simulink model "bh_explore_1dof_Newton_vs_Simscape"  (R2026b)
settings: Solver=ode15s  StopTime=30  MaxStep=0.001  RelTol=1e-5  EnableMultiTasking=on
undefined symbols (not defined in the file or in its folder): plant_T
settings Model: Creator=smiller  LastModifiedBy=bhorton
settings SolverCC: ZeroCrossAlgorithm=Adaptive
settings DataIOCC: LimitDataPoints=on  ReturnWorkspaceOutputs=off  SaveFormat=Array
settings OptimizationCC: LifeSpan=inf
settings DebuggingCC: AllowSymbolicDim=off  ArithmeticOperatorsInVariantConditions=warning  MergeDetectMultiDrivingBlocksExec=none  SFExecutionAtInitializationDiag=none  SFNoUnconditionalDefaultTransitionDiag=warning  SFUnexpectedBacktrackingDiag=warning  SolverPrmCheckMsg=warning  StateNameClashWarn=warning  UnderspecifiedInitializationDetection=Classic
settings HardwareCC: ProdEndianess=Unspecified  ProdHWDeviceType=32-bit Generic  ProdIntDivRoundTo=Undefined  ProdLargestAtomicFloat=None
settings ModelReferenceCC: PropagateSignalLabelsOutOfModel=off
settings SFSimCC: CustomCodeUndefinedFunction=UseInterfaceOnly  SimUseLocalCustomCode=off
settings RTWCC: DLArmComputeVersion=19.05  RTWUseLocalCustomCode=off
settings CodeAppCC: StateflowObjectComments=on
settings GRTTargetCC: TargetLangStandard=C89/C90 (ANSI)
settings ConfigComp: CovExternalEMLEnable=off  CovSFcnEnable=off  CovSaveCumulativeToWorkspaceVar=on  CovSaveSingleToWorkspaceVar=on
settings SimscapeCC: SimscapeNormalizeSystem=off  SimscapeUseEnergyAccounting=off
settings ExplorerConfigSet: InternalSimMechanicsExplorerSettings=|
  | <ExplorerConfiguration>
  | 
  |   <canonicalview>planar_xy</canonicalview>
  | 
  |   <TilePanel>
  |     <TileInfo>
  |       <Tiles Columns="2" Count="2" Height="500" Rows="1" Width="911">
  |         <Row Weight="1"/>
  |         <Column Weight="0.5"/>
  |         <Column Weight="0.5"/>
  |         <Tile Height="1" Width="1" X="0" Y="0"/>
  |         <Tile Height="1" Width="1" X="1" Y="0"/>
  |       </Tiles>
  |     </TileInfo>
  |     <SceneInfo>
  |       <SceneViewer>
  |         <IsThisViewStd>
  |           <IsStandardView>off</IsStandardView>
  |           <StandardViewName>Front</StandardViewName>
  |         </IsThisViewStd>
  |         <BGColor>
  |           <R>0.60000002384185791</R>
  |           <G>0.60000002384185791</G>
  |           <B>0.60000002384185791</B>
  |           <A>1</A>
  |         </BGColor>
  |         <Camera>
  |           <DoPerspective>off</DoPerspective>
  |           <Position>
  |             <X>-0.0052100000000000002</X>
  |             <Y>0.64158999999999999</Y>
  |             <Z>11.781499999999999</Z>
  |           </Position>
  |           <Center>
  |             <X>-0.0052100000000000002</X>
  |             <Y>0.64158999999999999</Y>
  |             <Z>1.5026299999999999</Z>
  |           </Center>
  |           <Up>
  |             <X>0</X>
  |             <Y>1</Y>
  |             <Z>0</Z>
  |           </Up>
  |           <XLim>0.92107080925589679</XLim>
  |           <YLim>0.92107080925589679</YLim>
  |           <ViewLimDist>0.01</ViewLimDist>
  |         </Camera>
  |       </SceneViewer>
  |       <SceneViewer>
  |         <IsThisViewStd>
  |           <IsStandardView>off</IsStandardView>
  |           <StandardViewName>Front</StandardViewName>
  |         </IsThisViewStd>
  |         <BGColor>
  |           <R>0.60000002384185791</R>
  |           <G>0.60000002384185791</G>
  |           <B>0.60000002384185791</B>
  |           <A>1</A>
  |         </BGColor>
  |         <Camera>
  |           <DoPerspective>off</DoPerspective>
  |           <Position>
  |             <X>3.9547400000000001</X>
  |             <Y>5.0512199999999998</Y>
  |             <Z>10.1366</Z>
  |           </Position>
  |           <Center>
  |             <X>0.44324999999999998</X>
  |             <Y>1.1275999999999999</Y>
  |             <Z>1.3108200000000001</Z>
  |           </Center>
  |           <Up>
  |             <X>-0.16378130891016329</X>
  |             <Y>0.92397727065044477</Y>
  |             <Z>-0.34560336539598169</Z>
  |           </Up>
  |           <XLim>0.80230735668277542</XLim>
  |           <YLim>0.80230735668277542</YLim>
  |           <ViewLimDist>0.01</ViewLimDist>
  |         </Camera>
  |       </SceneViewer>
  |     </SceneInfo>
  |   </TilePanel>
  | 
  |   <MechEditorPanel>
  |     <GfxPanelCameraMap/>
  |     <Cameras/>
  |     <VideoCreator>
  |       <IncludeTiles>All</IncludeTiles>
  |       <IncludeTime>on</IncludeTime>
  |       <IncludeWorldFrame>off</IncludeWorldFrame>
  |       <PlaybackSpeedRatio>4</PlaybackSpeedRatio>
  |       <FrameRate>30</FrameRate>
  |       <FrameSize>[400, 400]</FrameSize>
  |       <VideoFormat>UncompressedAVI</VideoFormat>
  |     </VideoCreator>
  |   </MechEditorPanel>
  | 
  |   <PlaybackSettings>
  |     <PlaybackSpeedFactor>1</PlaybackSpeedFactor>
  |   </PlaybackSettings>
  | 
  | </ExplorerConfiguration>

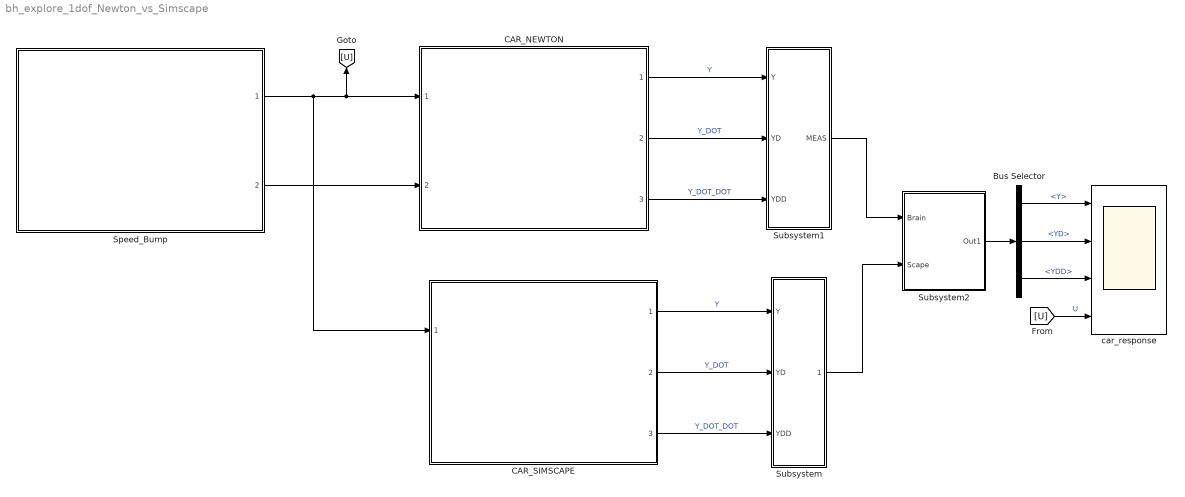
== system bh_explore_1dof_Newton_vs_Simscape ==
  Bus Selector : BusSelector  OutputSignals=Y,YD,YDD
  CAR_NEWTON : Subsystem  ReferencedSubsystem=bh_COMPONENT_1dof_NEWTON  m=plant_T.m  c=plant_T.c  k=plant_T.k  y0=IC_T.y  y_dot_0=IC_T.y_dot
  CAR_SIMSCAPE : Subsystem  ReferencedSubsystem=bh_COMPONENT_1dof_SIMSCAPE  m=plant_T.m  c=plant_T.c  k=plant_T.k  L_EQ=IC_T.L_EQ  U_m_rel_R=IC_T.U_m_rel_R  U_m_rel_R_dot=IC_T.U_m_rel_R_dot
  Speed_Bump : Subsystem  ReferencedSubsystem=bh_COMPONENT_U_rectangular_pulse
  Subsystem : Subsystem
  Subsystem1 : Subsystem
  Subsystem2 : Subsystem
  car_response : Scope  NumInputPorts=4
      settings: ActiveDisplayString=4  ActiveDisplayYMinimum=-0.018749999999999996  ActiveDisplayYMaximum=0.16874999999999998
  wires:
  CAR_SIMSCAPE/3 -> Subsystem/3(YDD)  "Y_DOT_DOT"
  CAR_SIMSCAPE/2 -> Subsystem/2(YD)  "Y_DOT"
  CAR_SIMSCAPE/1 -> Subsystem/1(Y)  "Y"
  [U] -> car_response/4  "U"
  Speed_Bump/1 -> CAR_SIMSCAPE/1, [U], CAR_NEWTON/1
  Speed_Bump/2 -> CAR_NEWTON/2
  Subsystem1/1(MEAS) -> Subsystem2/1(Brain)
  Bus Selector/3 -> car_response/3  "<YDD>"
  Subsystem/1(MEAS) -> Subsystem2/2(Scape)
  Bus Selector/1 -> car_response/1  "<Y>"
  Subsystem2/1(Out1) -> Bus Selector/1
  Bus Selector/2 -> car_response/2  "<YD>"
  CAR_NEWTON/1 -> Subsystem1/1(Y)  "Y"
  CAR_NEWTON/2 -> Subsystem1/2(YD)  "Y_DOT"
  CAR_NEWTON/3 -> Subsystem1/3(YDD)  "Y_DOT_DOT"

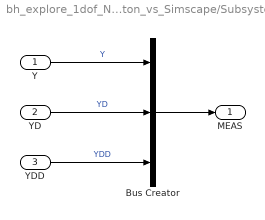
== system bh_explore_1dof_Newton_vs_Simscape/Subsystem ==
  Y : Inport
  YD : Inport  Port=2
  YDD : Inport  Port=3
  Bus Creator : BusCreator  Inputs=3
  MEAS : Outport
  wires:
  YD/1 -> Bus Creator/2  "YD"
  YDD/1 -> Bus Creator/3  "YDD"
  Y/1 -> Bus Creator/1  "Y"
  Bus Creator/1 -> MEAS/1

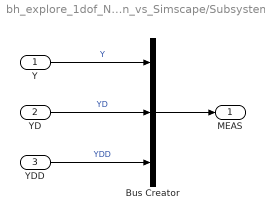
== system bh_explore_1dof_Newton_vs_Simscape/Subsystem1 ==
  Y : Inport
  YD : Inport  Port=2
  YDD : Inport  Port=3
  Bus Creator : BusCreator  Inputs=3
  MEAS : Outport
  wires:
  YD/1 -> Bus Creator/2  "YD"
  YDD/1 -> Bus Creator/3  "YDD"
  Y/1 -> Bus Creator/1  "Y"
  Bus Creator/1 -> MEAS/1

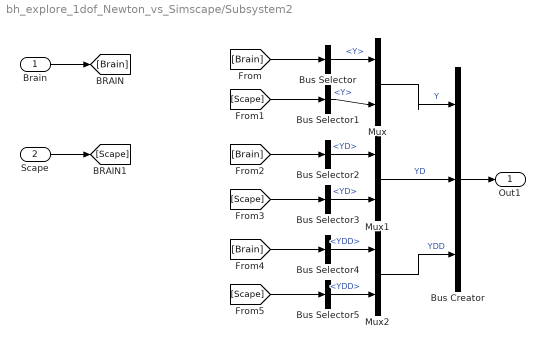
== system bh_explore_1dof_Newton_vs_Simscape/Subsystem2 ==
  Brain : Inport
  Scape : Inport  Port=2
  Bus Creator : BusCreator  Inputs=3
  Bus Selector : BusSelector  OutputSignals=Y
  Bus Selector1 : BusSelector  OutputSignals=Y
  Bus Selector2 : BusSelector  OutputSignals=YD
  Bus Selector3 : BusSelector  OutputSignals=YD
  Bus Selector4 : BusSelector  OutputSignals=YDD
  Bus Selector5 : BusSelector  OutputSignals=YDD
  Mux : Mux  Inputs=2
  Mux1 : Mux  Inputs=2
  Mux2 : Mux  Inputs=2
  Out1 : Outport
  wires:
  Scape/1 -> [Scape]
  Brain/1 -> [Brain]
  [Brain] -> Bus Selector/1
  [Scape] -> Bus Selector1/1
  Bus Selector/1 -> Mux/1  "<Y>"
  Bus Selector1/1 -> Mux/2  "<Y>"
  Bus Selector2/1 -> Mux1/1  "<YD>"
  [Brain] -> Bus Selector2/1
  [Scape] -> Bus Selector3/1
  Bus Selector3/1 -> Mux1/2  "<YD>"
  Bus Selector4/1 -> Mux2/1  "<YDD>"
  [Brain] -> Bus Selector4/1
  [Scape] -> Bus Selector5/1
  Bus Selector5/1 -> Mux2/2  "<YDD>"
  Mux1/1 -> Bus Creator/2  "YD"
  Mux/1 -> Bus Creator/1  "Y"
  Mux2/1 -> Bus Creator/3  "YDD"
  Bus Creator/1 -> Out1/1
